simulink model "A_1_VariableFrequencyOscillator"  (R2018b)
settings: Solver=VariableStepAuto  StartTime=0.0  StopTime=10.0  RelTol=1e-3
settings Model: Creator=Gowtham  LastModifiedBy=Gowtham

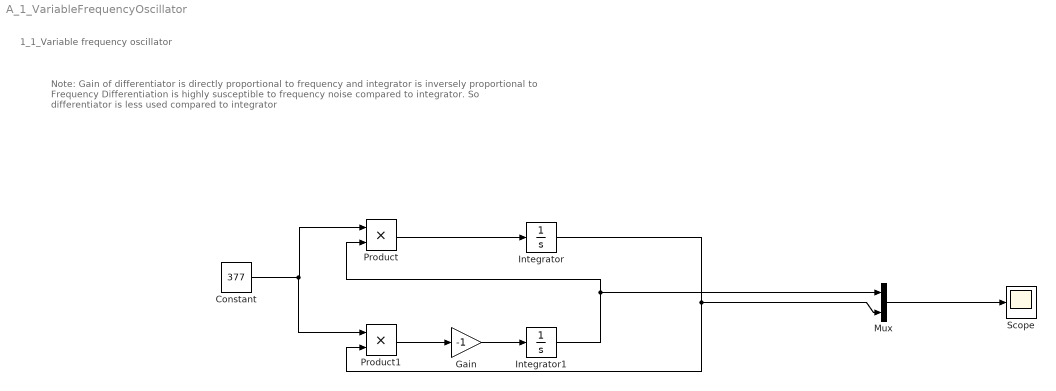
== system A_1_VariableFrequencyOscillator ==
  note: Note: Gain of differentiator is directly proportional to frequency and integrator is inversely proportional to Frequency
      | Differentiation is highly susceptible to frequency noise compared to integrator. So differentiator is less used compared to integrator
  note: 1_1_Variable frequency oscillator
  Constant : Constant  Value=377
  Gain : Gain  Gain=-1
  Integrator : Integrator  InitialCondition=1
  Integrator1 : Integrator  InitialCondition=1
  Mux : Mux  Inputs=2
  Product : Product
  Product1 : Product
  Scope : Scope
  wires:
  Product1/1 -> Gain/1
  Gain/1 -> Integrator1/1
  Product/1 -> Integrator/1
  Integrator1/1 -> Mux/1, Product/2
  Integrator/1 -> Mux/2, Product1/2
  Constant/1 -> Product1/1, Product/1
  Mux/1 -> Scope/1
